simulink model "SS_MMC_time_domain_small_signal"  (R2023b)
settings: Solver=VariableStepAuto  StartTime=0.0  StopTime=10.0  RelTol=1e-3
settings Model: Creator=dli313  LastModifiedBy=dongyuli

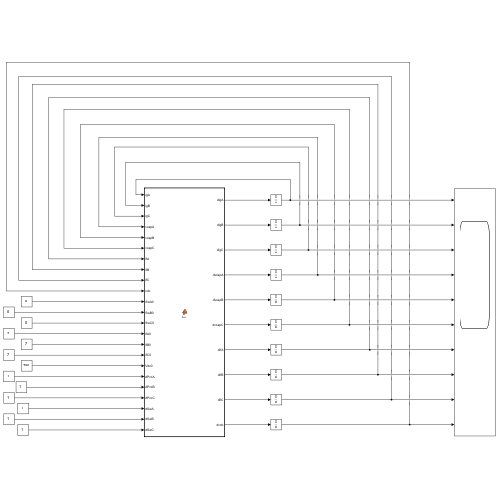
[thumbnail: Simulink's stored preview of the top-level diagram]
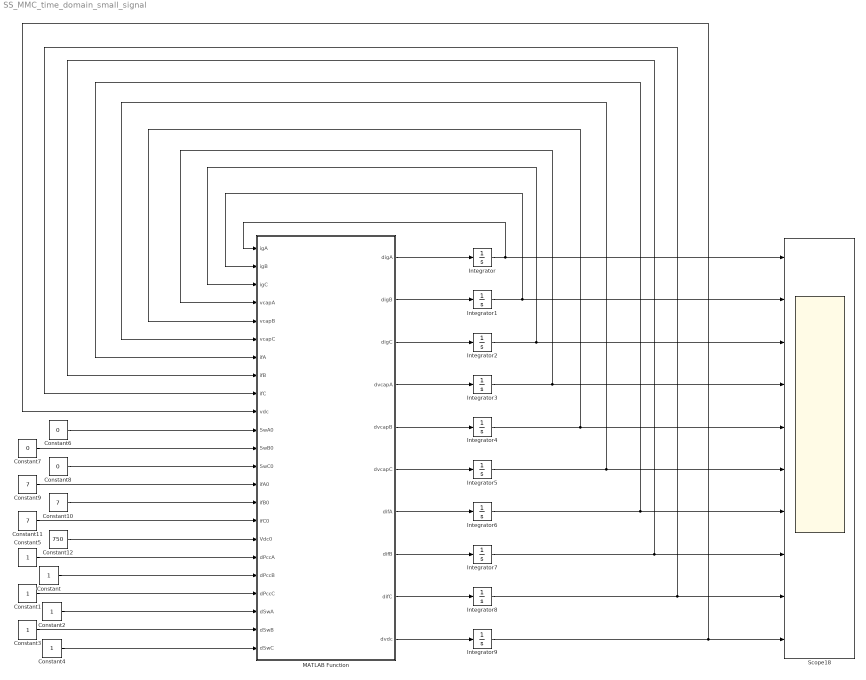
== system SS_MMC_time_domain_small_signal ==
  Constant{,1..5} (6 alike) : Constant
  Constant10 : Constant  Value=7
  Constant11 : Constant  Value=7
  Constant12 : Constant  Value=750
  Constant6 : Constant  Value=0
  Constant7 : Constant  Value=0
  Constant8 : Constant  Value=0
  Constant9 : Constant  Value=7
  Integrator{,1..9} (10 alike) : Integrator
  MATLAB Function : MATLAB Function  TreatAsAtomicUnit=on
  Scope18 : Scope  NumInputPorts=10
  wires:
  MATLAB Function/1(digA) -> Integrator/1
  MATLAB Function/2(digB) -> Integrator1/1
  MATLAB Function/3(digC) -> Integrator2/1
  MATLAB Function/4(dvcapA) -> Integrator3/1
  MATLAB Function/5(dvcapB) -> Integrator4/1
  MATLAB Function/6(dvcapC) -> Integrator5/1
  MATLAB Function/7(difA) -> Integrator6/1
  MATLAB Function/8(difB) -> Integrator7/1
  MATLAB Function/9(difC) -> Integrator8/1
  MATLAB Function/10(dvdc) -> Integrator9/1
  Integrator/1 -> Scope18/1, MATLAB Function/1(igA)
  Integrator1/1 -> Scope18/2, MATLAB Function/2(igB)
  Integrator2/1 -> Scope18/3, MATLAB Function/3(igC)
  Integrator3/1 -> Scope18/4, MATLAB Function/4(vcapA)
  Integrator4/1 -> Scope18/5, MATLAB Function/5(vcapB)
  Integrator5/1 -> Scope18/6, MATLAB Function/6(vcapC)
  Integrator6/1 -> Scope18/7, MATLAB Function/7(ifA)
  Integrator8/1 -> Scope18/9, MATLAB Function/9(ifC)
  Integrator9/1 -> Scope18/10, MATLAB Function/10(vdc)
  Integrator7/1 -> Scope18/8, MATLAB Function/8(ifB)
  Constant6/1 -> MATLAB Function/11(SwA0)
  Constant7/1 -> MATLAB Function/12(SwB0)
  Constant8/1 -> MATLAB Function/13(SwC0)
  Constant9/1 -> MATLAB Function/14(ifA0)
  Constant10/1 -> MATLAB Function/15(ifB0)
  Constant11/1 -> MATLAB Function/16(ifC0)
  Constant12/1 -> MATLAB Function/17(Vdc0)
  Constant2/1 -> MATLAB Function/21(dSwA)
  Constant/1 -> MATLAB Function/19(dPccB)
  Constant3/1 -> MATLAB Function/22(dSwB)
  Constant1/1 -> MATLAB Function/20(dPccC)
  Constant4/1 -> MATLAB Function/23(dSwC)
  Constant5/1 -> MATLAB Function/18(dPccA)

== matlab function SS_MMC_time_domain_small_signal/MATLAB Function ==
  data: igA input; digA output; igB input; igC input; vcapA input; vcapB input; vcapC input; ifA input; ifB input; ifC input; vdc input; SwA0 input; SwB0 input; SwC0 input; ifA0 input; ifB0 input; ifC0 input; Vdc0 input; digB output; digC output; dvcapA output; dvcapB output; dvcapC output; difA output; difB output; difC output; dvdc output; dPccA input; dPccB input; dPccC input; dSwA input; dSwB input; dSwC input
function [digA, digB, digC, dvcapA, dvcapB, dvcapC, difA, difB, difC, dvdc] = fcn(igA, igB, igC, vcapA, vcapB, vcapC, ifA, ifB, ifC, vdc, SwA0, SwB0, SwC0, ifA0, ifB0, ifC0, Vdc0, dPccA, dPccB, dPccC, dSwA, dSwB, dSwC)

RgA = 1;
RgB = 1;
RgC = 1;

RfA = 0.5;
RfB = 0.5;
RfC = 0.5;

RcfA = 0.5;
RcfB = 0.5;
RcfC = 0.5;

LgA = 3.3e-3;
LgB = 3.3e-3;
LgC = 3.3e-3;

LfA = 6.25e-3;
LfB = 6.25e-3;
LfC = 6.25e-3;

CfA = 94e-6;
CfB = 94e-6;
CfC = 94e-6;

Rdc = 0.01;
Cdc = 450e-6;

A = [(-RgA-RcfA)/LgA 0 0 -1/LgA 0 0 RcfA/LgA 0 0 0;
     0 (-RgB-RcfB)/LgB 0 0 -1/LgB 0 0 RcfB/LgB 0 0;
     0 0 (-RgC-RcfC)/LgC 0 0 -1/LgC 0 0 RcfC/LgC 0;
     1/CfA 0 0 0 0 0 -1/CfA 0 0 0;
     0 1/CfA 0 0 0 0 0 -1/CfB 0 0;
     0 0 1/CfC 0 0 0 0 0 -1/CfC 0;
     RcfA 0 0 1/LfA 0 0 (-RcfA-RfA)/LfA 0 0 -SwA0/LfA;
     0 RcfB/LfB 0 0 1/LfB 0 0 (-RfB-RfB)/LfB 0 -SwB0/LfB;
     0 0 RcfC/LfC 0 0 1/LfC 0 0 (-RcfC-RfC)/LfC -SwC0/LfC;
     0 0 0 0 0 0 SwA0/Cdc SwB0/Cdc SwC0/Cdc -1/(Rdc*Cdc)];

B = [1/LgA 0 0 0 0 0;
    0 1/LgB 0 0 0 0;
    0 0 1/LgC 0 0 0;
    0 0 0 0 0 0;
    0 0 0 0 0 0;
    0 0 0 0 0 0;
    0 0 0 -Vdc0/LfA 0 0;
    0 0 0 0 -Vdc0/LfB 0;
    0 0 0 0 0 -Vdc0/LfC;
    0 0 0 ifA0/Cdc ifB0/Cdc ifC0/Cdc];

X = [igA, igB, igC, vcapA, vcapB, vcapC, ifA, ifB, ifC, vdc]';

U = [dPccA, dPccB, dPccC, dSwA, dSwB, dSwC]';

dX = A*X + B*U;

digA = dX(1);
digB = dX(2);
digC = dX(3);
dvcapA = dX(4);
dvcapB = dX(5);
dvcapC = dX(6);
difA = dX(7);
difB = dX(8);
difC = dX(9);
dvdc = dX(10);

end
